simulink model "ztrack"  (R2020b)
settings: Solver=VariableStepAuto  StartTime=0.0  StopTime=50  RelTol=1e-3
libraries: simulink x1
settings Model: Creator=sumit  LastModifiedBy=sumit

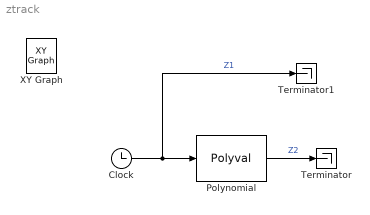
== system ztrack ==
  Clock : Clock
  Polynomial : Polyval  Coefs=[-0.002 0.1 0.1 0]
  Terminator : Terminator
  Terminator1 : Terminator
  XY Graph : simulink/Sinks/XY Graph  IOType=viewer  xmin=0  xmax=50  ymin=0  ymax=50  st=-1
  wires:
  Polynomial/1 -> Terminator/1  "Z2"
  Clock/1 -> Terminator1/1, Polynomial/1  "Z1"
